simulink model "Exp5_simulink"  (R2022a)
settings: Solver=VariableStepAuto  StartTime=0.0  StopTime=1  RelTol=1e-3
values from neighbouring files (symbols this model uses):
  Pm = Pe    (= 0.9)    [Exp5.m]
  Pm2 = Eg*V/x2    (= 0.88)    [Exp5.m]
  Pm3 = Eg*V/x3    (= 2)    [Exp5.m]
settings Model: Creator=admin  LastModifiedBy=supreeth
settings SolverCC: AlgebraicLoopSolver=TrustRegion
settings DebuggingCC: UnconnectedInputMsg=warning  UnconnectedOutputMsg=warning  UnconnectedLineMsg=warning  SFMachineParentedDataDiag=warning

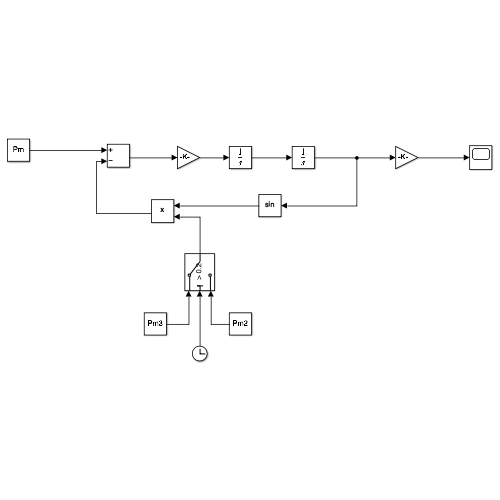
[thumbnail: Simulink's stored preview of the top-level diagram]
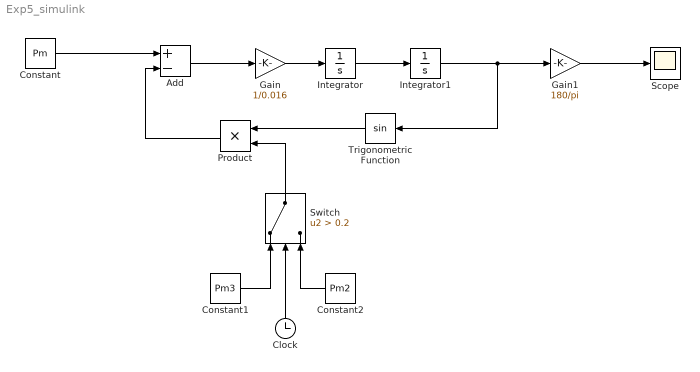
== system Exp5_simulink ==
  Add : Sum  Inputs=+-
  Clock : Clock
  Constant : Constant  Value=Pm
  Constant1 : Constant  Value=Pm3
  Constant2 : Constant  Value=Pm2
  Gain : Gain  Gain=1/0.016
  Gain1 : Gain  Gain=180/pi
  Integrator : Integrator
  Integrator1 : Integrator
  Product : Product
  Scope : Scope
  Switch : Switch  Criteria=u2 > Threshold  Threshold=0.2  SaturateOnIntegerOverflow=off  InputSameDT=off
  Trigonometric Function : Trigonometry
  wires:
  Constant1/1 -> Switch/1
  Clock/1 -> Switch/2
  Constant2/1 -> Switch/3
  Constant/1 -> Add/1
  Add/1 -> Gain/1
  Gain/1 -> Integrator/1
  Integrator/1 -> Integrator1/1
  Integrator1/1 -> Trigonometric Function/1, Gain1/1
  Switch/1 -> Product/2
  Product/1 -> Add/2
  Trigonometric Function/1 -> Product/1
  Gain1/1 -> Scope/1
